simulink model "TP"  (R2016a)
settings: Solver=VariableStepAuto  SolverMode=SingleTasking  StartTime=0.0  StopTime=10  RelTol=1e-3
values from neighbouring files (symbols this model uses):
  F1 = -acker(A,B,P1)    [Data.m]    (also in Q5.m)
  K1 = acker(A',C',Po1)'    [Data.m]    (also in Q5.m)
undefined symbols (not defined in the file or in its folder): A, B, C, Kstatique
libraries: cstblocks x3
settings Model: Creator=hnadour2017  LastModifiedBy=NAD
settings DebuggingCC: SFUnexpectedBacktrackingDiag=error  SFNoUnconditionalDefaultTransitionDiag=error
settings GRTTargetCC: TargetLangStandard=C99 (ISO)  GeneratePreprocessorConditionals=Use local settings
settings ConfigComp: CovMetricSettings=dwe  CovHtmlReporting=off  CovSaveCumulativeToWorkspaceVar=off  CovSaveSingleToWorkspaceVar=off  CovExternalEMLEnable=on

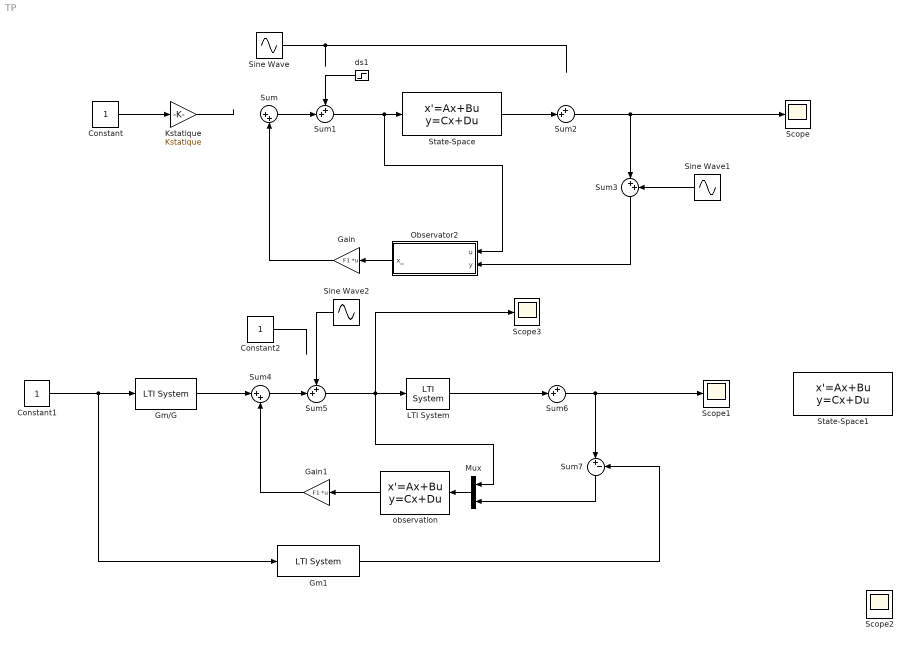
== system TP ==
  Constant : Constant
  Constant1 : Constant
  Constant2 : Constant
  Gain : Gain  Gain=F1  Multiplication=Matrix(K*u) (u vector)
  Gain1 : Gain  Gain=F1  Multiplication=Matrix(K*u) (u vector)
  Gm/G : cstblocks/LTI System  sys=Gm/G/K1_  IC=[]
  Gm1 : cstblocks/LTI System  sys=Gm  IC=[]
  Kstatique : Gain  Gain=Kstatique
  LTI System : cstblocks/LTI System  sys=G  IC=[]
  Mux : Mux  Inputs=2
  Observator2 : Subsystem
  Scope{,1..3} (4 alike) : Scope
  Sine Wave : Sin  Amplitude=0.1  Frequency=0.05  SampleTime=0
  Sine Wave1 : Sin  Amplitude=0.1  Frequency=100  SampleTime=0
  Sine Wave2 : Sin  Amplitude=100  Frequency=1000  SampleTime=0
  State-Space : StateSpace  A=A  B=B  C=C  D=0  X0=0
  State-Space1 : StateSpace  A=A  B=B  C=C  D=0  X0=0
  Sum : Sum  Inputs=|++
  Sum{1..2,5..6} (4 alike) : Sum  Inputs=++|
  Sum3 : Sum  Inputs=|++
  Sum4 : Sum  Inputs=|++
  Sum7 : Sum  Inputs=|+-
  ds1 : Step  Time=3  SampleTime=0
  observation : StateSpace  A=A-K1*C  B=[B , K1]  C=eye(3,3)  D=zeros(3,2)  X0=0
  wires:
  Sum1/1 -> Observator2/1(u), State-Space/1
  Observator2/1(x_) -> Gain/1
  Gain/1 -> Sum/2
  Constant/1 -> Kstatique/1
  Sum/1 -> Sum1/2
  State-Space/1 -> Sum2/2
  Sum2/1 -> Sum3/1, Scope/1
  Sum3/1 -> Observator2/2(y)
  Sine Wave/1 -> ?
  Sine Wave1/1 -> Sum3/2
  Sum5/1 -> Mux/1, LTI System/1, Scope3/1
  observation/1 -> Gain1/1
  Gain1/1 -> Sum4/2
  Sum4/1 -> Sum5/2
  LTI System/1 -> Sum6/2
  Sum7/1 -> Mux/2
  Sine Wave2/1 -> Sum5/1
  ? -> ?
  Kstatique/1 -> ?
  Sum6/1 -> Sum7/1, Scope1/1
  Constant1/1 -> Gm1/1, Gm/G/1
  Gm/G/1 -> Sum4/1
  Gm1/1 -> Sum7/2
  Mux/1 -> observation/1
  Constant2/1 -> ?
  ds1/1 -> Sum1/1

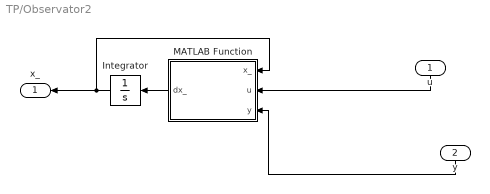
== system TP/Observator2 ==
  u : Inport
  y : Inport  Port=2
  Integrator : Integrator  InitialCondition=[0;0;0]
  MATLAB Function : MATLAB Function  TreatAsAtomicUnit=on
  x_ : Outport
  wires:
  Integrator/1 -> MATLAB Function/1(x_), x_/1
  MATLAB Function/1(dx_) -> Integrator/1
  u/1 -> MATLAB Function/2(u)
  y/1 -> MATLAB Function/3(y)

== matlab function TP/Observator2/MATLAB Function ==
  data: x_ input; u input; dx_ output; y input
function dx_=fct(x_,u,y)

A =[
  -8.0000   -2.6250   -2.2500
    8.0000         0         0
         0    1.0000         0];

    B =[
     4
     0
     0  ];
 C=[0    1.0938    5.4688];
 K1=[52.9143
     47.5429
     0.9143];

 dx_=(A-K1*C)*x_+B*u+K1*y;
